simulink model "velo_pi"  (R2019a)
settings: Solver=FixedStepAuto  StartTime=0.0  StopTime=10.0  RelTol=1e-3  EnableMultiTasking=on
values from neighbouring files (symbols this model uses):
  ts = 1/50    (= 0.02)    [sim_init.m]    (also in sim_param.mat; velo_id_tc.m; velo_pi_mdb.m)
libraries: arduinolib x3
settings Model: ExtModeTrigDuration=2  Creator=Daichi  LastModifiedBy=Daichi
settings OptimizationCC: EnhancedBackFolding=on  PassReuseOutputArgsAs=Individual arguments  MaxStackSize=64  OptimizeBlockOrder=speed  DifferentSizesBufferReuse=on  OptimizationCustomize=off
settings DebuggingCC: ParameterTunabilityLossMsg=error
settings HardwareCC: ProdBitPerInt=16  ProdBitPerPointer=16  ProdBitPerSizeT=16  ProdBitPerPtrDiffT=16  ProdLargestAtomicFloat=None  ProdWordSize=8  ProdHWDeviceType=Atmel->AVR  UseEmbeddedCoderFeatures=off
settings SFSimCC: MATLABDynamicMemAlloc=off
settings RTWCC: SystemTargetFile=ert.tlc  HardwareBoard=Arduino Mega 2560  TLCOptions=-aInlineSetEventsForThisBaseRateFcn=TLC_FALSE -aSuppressMultiTaskScheduler=TLC_FALSE -aRateBasedStepFcn=1  TemplateMakefile=ert_default_tmf  GenerateReport=on  Toolchain=Arduino AVR  BuildConfiguration=Faster Runs  IncludeHyperlinkInReport=on  LaunchReport=on  GenerateTraceInfo=on  GenerateTraceReport=on  GenerateTraceReportSl=on  GenerateTraceReportSf=on  GenerateTraceReportEml=on
settings CodeAppCC: ForceParamTrailComments=on  IgnoreCustomStorageClasses=off  OperatorAnnotations=on  SimulinkDataObjDesc=on  SFDataObjDesc=on  InsertBlockDesc=on
settings ERTTargetCC: SupportContinuousTime=on  SupportNonInlinedSFcns=on  SupportVariableSizeSignals=on  ExtModeStaticAllocSize=2048

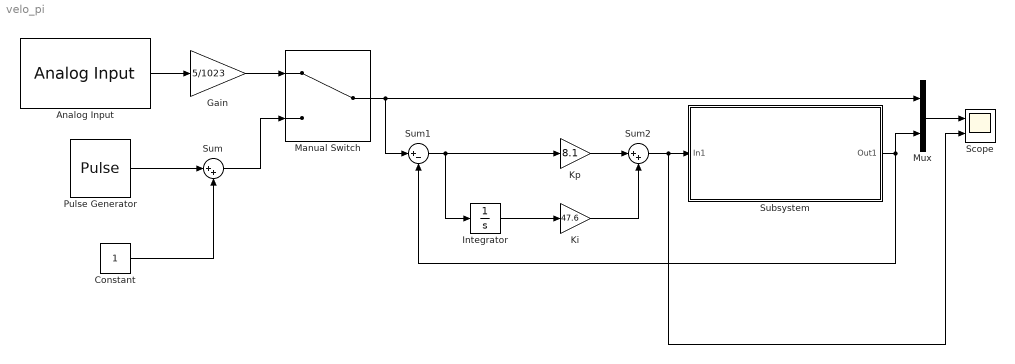
== system velo_pi ==
  Analog Input : arduinolib/Analog Input  pinNumber=1  ReadResultsOnly=off  ConversionTriggerSource=Software  ExternalTriggerType=uint32(0)  OutputDataType=uint16  EnableConversionCompleteNotify=off  EnableOuputStatus=off  SampleTime=1/50  blockPlatform=arduino
  Constant : Constant
  Gain : Gain  Gain=5/1023  OutDataTypeStr=double
  Integrator : Integrator
  Ki : Gain  Gain=47.6  OutDataTypeStr=double
  Kp : Gain  Gain=8.1  OutDataTypeStr=double
  Manual Switch : ManualSwitch
  Mux : Mux  Inputs=2
  Pulse Generator : DiscretePulseGenerator  Amplitude=0.5  Period=10/ts  PulseWidth=5/ts  PhaseDelay=50  SampleTime=ts
  Scope : Scope  NumInputPorts=2
  Subsystem : Subsystem
  Sum : Sum  Inputs=|++
  Sum1 : Sum  Inputs=|+-
  Sum2 : Sum  Inputs=|++
  wires:
  Pulse Generator/1 -> Sum/1
  Ki/1 -> Sum2/2
  Constant/1 -> Sum/2
  Sum2/1 -> Scope/2, Subsystem/1(In1)
  Kp/1 -> Sum2/1
  Sum/1 -> Manual Switch/2
  Integrator/1 -> Ki/1
  Gain/1 -> Manual Switch/1
  Mux/1 -> Scope/1
  Subsystem/1(Out1) -> Sum1/2, Mux/2
  Analog Input/1 -> Gain/1
  Sum1/1 -> Integrator/1, Kp/1
  Manual Switch/1 -> Sum1/1, Mux/1

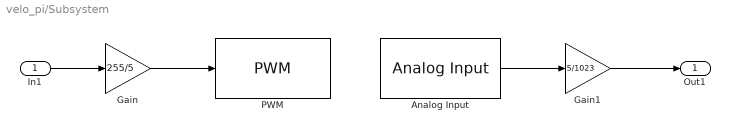
== system velo_pi/Subsystem ==
  In1 : Inport
  Analog Input : arduinolib/Analog Input  pinNumber=0  ReadResultsOnly=off  ConversionTriggerSource=Software  ExternalTriggerType=uint32(0)  OutputDataType=uint16  EnableConversionCompleteNotify=off  EnableOuputStatus=off  SampleTime=ts  blockPlatform=arduino
  Gain : Gain  Gain=255/5  OutDataTypeStr=double
  Gain1 : Gain  Gain=5/1023  OutDataTypeStr=double
  PWM : arduinolib/PWM  pinNumber=3  EnableInputFrequency=off  InitialFrequency=2000  InitialDutyCycle=0  NotificationType=None  blockPlatform=arduino
  Out1 : Outport  OutDataTypeStr=double
  wires:
  In1/1 -> Gain/1
  Analog Input/1 -> Gain1/1
  Gain/1 -> PWM/1
  Gain1/1 -> Out1/1
